simulink model "FP_Solutions_Part_2_torque_free"  (R2022a)
settings: Solver=FixedStepAuto  StartTime=0.0  StopTime=orbital_period  FixedStep=10  RelTol=1e-3
values from neighbouring files (symbols this model uses):
  E_b_ECI_0 = C2EulerAngles(C_b_ECI_0)    [FP3_Disturbances_RS.m]
  J = [812.0396             0             0 ... (first row only)    [FP3_Disturbances_RS.m]
  q_b_ECI_0 = rotm2quat(C_b_ECI_0)    [FP3_Disturbances_RS.m]
  w_b_ECI_0 = [0.001; -0.001; 0.002]    [FP3_Disturbances_RS.m]
undefined symbols (not defined in the file or in its folder): T
settings Model: Creator=emehiel  LastModifiedBy=emehiel
settings SolverCC: AlgebraicLoopSolver=TrustRegion
settings DebuggingCC: UnconnectedInputMsg=warning  UnconnectedOutputMsg=warning  UnconnectedLineMsg=warning  SFMachineParentedDataDiag=warning

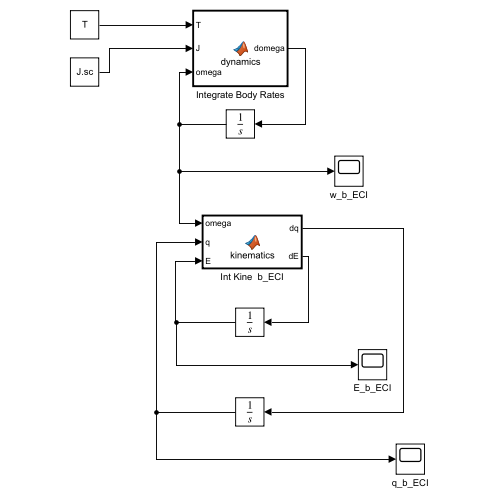
[thumbnail: Simulink's stored preview of the top-level diagram]
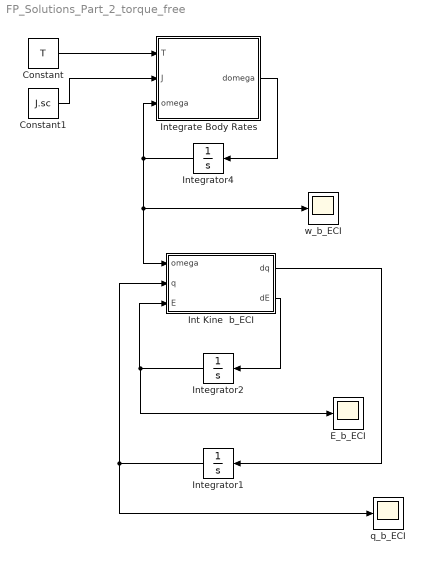
== system FP_Solutions_Part_2_torque_free ==
  Constant : Constant  Value=T
  Constant1 : Constant  Value=J.sc
  E_b_ECI : Scope
  Int Kine  b_ECI : MATLAB Function  TreatAsAtomicUnit=on
  Integrate Body Rates : MATLAB Function  TreatAsAtomicUnit=on
  Integrator1 : Integrator  InitialCondition=q_b_ECI_0
  Integrator2 : Integrator  InitialCondition=E_b_ECI_0
  Integrator4 : Integrator  InitialCondition=w_b_ECI_0
  q_b_ECI : Scope
  w_b_ECI : Scope
  wires:
  Constant/1 -> Integrate Body Rates/1(T)
  Constant1/1 -> Integrate Body Rates/2(J)
  Integrate Body Rates/1(domega) -> Integrator4/1
  Integrator4/1 -> w_b_ECI/1, Int Kine  b_ECI/1(omega), Integrate Body Rates/3(omega)
  Integrator2/1 -> E_b_ECI/1, Int Kine  b_ECI/3(E)
  Integrator1/1 -> q_b_ECI/1, Int Kine  b_ECI/2(q)
  Int Kine  b_ECI/2(dE) -> Integrator2/1
  Int Kine  b_ECI/1(dq) -> Integrator1/1

== matlab function FP_Solutions_Part_2_torque_free/Int Kine  b_ECI ==
  data: omega input; q input; dq output; E input; dE output
function [dq,dE] = kinematics(omega, q, E)
%#codegen

% unpack quaternion

epsilon = q(1:3,1);
eta = q(4,1);

depsilon = 1/2*(eta*eye(3) + vect2cross(epsilon))*omega;
deta = -1/2*epsilon'*omega;

dq = [depsilon; deta];

LBI = 1/cos(E(2))*[cos(E(2)) sin(E(1))*sin(E(2))  cos(E(1))*sin(E(2));
                   0         cos(E(1))*cos(E(2)) -sin(E(1))*cos(E(2));
                   0         sin(E(1))            cos(E(1))];

dE = LBI*omega;

== matlab function FP_Solutions_Part_2_torque_free/Integrate Body Rates ==
  data: T input; J input; omega input; domega output
function domega = dynamics(T, J, omega)
%#codegen

domega = J\(T - cross(omega, J*omega));
